simulink model "dynamicsquat_2022a"  (R2022a)
settings: Solver=VariableStepAuto  StartTime=0.0  StopTime=stoptimetotal  RelTol=1e-3
values from neighbouring files (symbols this model uses):
  battery = load('params/battery_Tattu.mat').battery    [runsimulation.m]
  IC = load('params/initialcond/IC_HoverAt30mOcto.mat').IC    [runsimulation.m]
  maxleashvelocity = speed    [runsimulation.m]
  Motor = load('params/KDE4213XF-360_performancedata.mat').Motor    [runsimulation.m]
  motormult = motormults(:)    [runsimulation.m]
  octomodel = load('params/TarotT18.mat').octomodel    [runsimulation.m]
  saturationrpm = saturationrpms(:)    [runsimulation.m]
  scurvetimes = tvec'    [runsimulation.m]
  turbenabled = turb_idx-1    [runsimulation.m]
  velprofileX = qd(1,:)'    [runsimulation.m]
  velprofileY = qd(2,:)'    [runsimulation.m]
  windx = smallestwind + (largestwind-smallestwind)*rand    [runsimulation.m]
  windy = smallestwind + (largestwind-smallestwind)*rand    [runsimulation.m]
  windz = 0    [runsimulation.m]
  xref = xyzref(waypts,1)    [runsimulation.m]
  yref = xyzref(waypts,2)    [runsimulation.m]
undefined symbols (not defined in the file or in its folder): deg, DiscIntNeverNeededParam, F, Light, MIL, rad, s
libraries: aerolibconvert2 x2, shared6dof x1, aerolibwind2 x1
(part 2 of 2)

== system dynamicsquat_2022a/Motors/DC Motor 8/Mechanical part ==
  Static Friction Torque : Inport
  Electrical Torque : Inport  Port=2
  1/J Inertia constant : Gain  Gain=1/Motor.J
  "Df viscous damping coefficient Dynamic Friction coefficient " : Gain  Gain=Motor.Df
  Discrete-Time Integrator : DiscreteIntegrator  gainval=1  InitialCondition=IC.w8  SampleTime=octomodel.sampletime  ICPrevOutput=DiscIntNeverNeededParam  ICPrevScaledInput=DiscIntNeverNeededParam
  Sum1 : Sum  Inputs=--+-
  torque and thrust calculation : Subsystem
  w angular speed : Outport  VectorParamsAs1DForOutWhenUnconnected=off
  Thrust : Outport  Port=2  VectorParamsAs1DForOutWhenUnconnected=off
  Torque : Outport  Port=3  VectorParamsAs1DForOutWhenUnconnected=off
  wires:
  torque and thrust calculation/1(torque) -> Torque/1, Sum1/1
  torque and thrust calculation/2(thrusth) -> Thrust/1
  Electrical Torque/1 -> Sum1/3
  Sum1/1 -> 1/J Inertia constant/1
  Discrete-Time Integrator/1 -> "Df viscous damping coefficient Dynamic Friction coefficient "/1, torque and thrust calculation/1(w angular speed), w angular speed/1  "w angular speed"
  "Df viscous damping coefficient Dynamic Friction coefficient "/1 -> Sum1/4
  Static Friction Torque/1 -> Sum1/2
  1/J Inertia constant/1 -> Discrete-Time Integrator/1

== system dynamicsquat_2022a/Motors/DC Motor 1/Mechanical part/torque and thrust calculation ==
  w angular speed : Inport
  Convert rad/s to rmp : Gain  Gain=60/(2*pi)
  "Propeller model " : MATLAB Function  TreatAsAtomicUnit=on
  torque : Outport  VectorParamsAs1DForOutWhenUnconnected=off
  thrusth : Outport  Port=2  VectorParamsAs1DForOutWhenUnconnected=off
  wires:
  Convert rad/s to rmp/1 -> "Propeller model "/1(rpm)
  w angular speed/1 -> Convert rad/s to rmp/1
  "Propeller model "/2(thrust) -> thrusth/1
  "Propeller model "/1(torque) -> torque/1

== system dynamicsquat_2022a/Motors/DC Motor 2/Mechanical part/torque and thrust calculation ==
  w angular speed : Inport
  Convert rad/s to rmp : Gain  Gain=60/(2*pi)
  "Propeller model " : MATLAB Function  TreatAsAtomicUnit=on
  torque : Outport  VectorParamsAs1DForOutWhenUnconnected=off
  thrusth : Outport  Port=2  VectorParamsAs1DForOutWhenUnconnected=off
  wires:
  "Propeller model "/1(torque) -> torque/1
  "Propeller model "/2(thrust) -> thrusth/1
  w angular speed/1 -> Convert rad/s to rmp/1
  Convert rad/s to rmp/1 -> "Propeller model "/1(rpm)

== system dynamicsquat_2022a/Motors/DC Motor 3/Mechanical part/torque and thrust calculation ==
  w angular speed : Inport
  Convert rad/s to rmp : Gain  Gain=60/(2*pi)
  "Propeller model " : MATLAB Function  TreatAsAtomicUnit=on
  torque : Outport  VectorParamsAs1DForOutWhenUnconnected=off
  thrusth : Outport  Port=2  VectorParamsAs1DForOutWhenUnconnected=off
  wires:
  Convert rad/s to rmp/1 -> "Propeller model "/1(rpm)
  w angular speed/1 -> Convert rad/s to rmp/1
  "Propeller model "/2(thrust) -> thrusth/1
  "Propeller model "/1(torque) -> torque/1

== system dynamicsquat_2022a/Motors/DC Motor 4/Mechanical part/torque and thrust calculation ==
  w angular speed : Inport
  Convert rad/s to rmp : Gain  Gain=60/(2*pi)
  "Propeller model " : MATLAB Function  TreatAsAtomicUnit=on
  torque : Outport  VectorParamsAs1DForOutWhenUnconnected=off
  thrusth : Outport  Port=2  VectorParamsAs1DForOutWhenUnconnected=off
  wires:
  "Propeller model "/1(torque) -> torque/1
  "Propeller model "/2(thrust) -> thrusth/1
  w angular speed/1 -> Convert rad/s to rmp/1
  Convert rad/s to rmp/1 -> "Propeller model "/1(rpm)

== system dynamicsquat_2022a/Motors/DC Motor 5/Mechanical part/torque and thrust calculation ==
  w angular speed : Inport
  Convert rad/s to rmp : Gain  Gain=60/(2*pi)
  "Propeller model " : MATLAB Function  TreatAsAtomicUnit=on
  torque : Outport  VectorParamsAs1DForOutWhenUnconnected=off
  thrusth : Outport  Port=2  VectorParamsAs1DForOutWhenUnconnected=off
  wires:
  Convert rad/s to rmp/1 -> "Propeller model "/1(rpm)
  w angular speed/1 -> Convert rad/s to rmp/1
  "Propeller model "/2(thrust) -> thrusth/1
  "Propeller model "/1(torque) -> torque/1

== system dynamicsquat_2022a/Motors/DC Motor 6/Mechanical part/torque and thrust calculation ==
  w angular speed : Inport
  Convert rad/s to rmp : Gain  Gain=60/(2*pi)
  "Propeller model " : MATLAB Function  TreatAsAtomicUnit=on
  torque : Outport  VectorParamsAs1DForOutWhenUnconnected=off
  thrusth : Outport  Port=2  VectorParamsAs1DForOutWhenUnconnected=off
  wires:
  "Propeller model "/1(torque) -> torque/1
  "Propeller model "/2(thrust) -> thrusth/1
  w angular speed/1 -> Convert rad/s to rmp/1
  Convert rad/s to rmp/1 -> "Propeller model "/1(rpm)

== system dynamicsquat_2022a/Motors/DC Motor 7/Mechanical part/torque and thrust calculation ==
  w angular speed : Inport
  Convert rad/s to rmp : Gain  Gain=60/(2*pi)
  "Propeller model " : MATLAB Function  TreatAsAtomicUnit=on
  torque : Outport  VectorParamsAs1DForOutWhenUnconnected=off
  thrusth : Outport  Port=2  VectorParamsAs1DForOutWhenUnconnected=off
  wires:
  Convert rad/s to rmp/1 -> "Propeller model "/1(rpm)
  w angular speed/1 -> Convert rad/s to rmp/1
  "Propeller model "/2(thrust) -> thrusth/1
  "Propeller model "/1(torque) -> torque/1

== system dynamicsquat_2022a/Motors/DC Motor 8/Mechanical part/torque and thrust calculation ==
  w angular speed : Inport
  Convert rad/s to rmp : Gain  Gain=60/(2*pi)
  "Propeller model " : MATLAB Function  TreatAsAtomicUnit=on
  torque : Outport  VectorParamsAs1DForOutWhenUnconnected=off
  thrusth : Outport  Port=2  VectorParamsAs1DForOutWhenUnconnected=off
  wires:
  "Propeller model "/1(torque) -> torque/1
  "Propeller model "/2(thrust) -> thrusth/1
  w angular speed/1 -> Convert rad/s to rmp/1
  Convert rad/s to rmp/1 -> "Propeller model "/1(rpm)

== matlab function dynamicsquat_2022a/Motors/DC Motor 8/Mechanical part/torque and thrust calculation/Propeller model  ==
  data: torque output; rpm input; thrust output
function [torque,thrust] = fcn(rpm)
%% Tarot model data

%coefficient of thrust, empirically derived
coef_t = 0.065;
%thrust = coef_t * density of air * velocity^2 * propeller diameter (m) ^4
%velocity in rev/sec, where  1 rev/sec = 1 rpm/60
thrust = coef_t*1.225*(rpm/60)^2*.47^4; % 18.5 inches ~ 0.47 m
% empirically derived
torque = (2.138e-08)*rpm^2 + (-1.279e-05)*rpm ;% (0.0216);

end

== matlab function dynamicsquat_2022a/arrival condition ==
  data: currentpos input; arrived output; dest input
function arrived = fcn(currentpos,dest)
result=norm(currentpos-dest);
if result<2 % less than one meter from the goal
    arrived=1;
else
    arrived=0;
end

== matlab function dynamicsquat_2022a/Power Consumption Calculation ==
  data: DC input; tot_mot_i output; Imot input
function tot_mot_i  = fcn(DC,Imot)
imot=zeros(8,1);
for i=1:length(DC)
    imot(i)=DC(i)*Imot(i);
end
tot_mot_i=sum(imot);
tot_mot_i=sum(Imot);
end

== matlab function dynamicsquat_2022a/Drag Force and Moment Calculation ==
  data: Vw_nom input; Fdrag output; Vw_turb input; Vb input; wb input; Mdrag output; Eul input; windspecs parameter
function [Fdrag,Mdrag]  = fcn(Vw_nom,Vw_turb,Vb,wb,Eul, windspecs)
%% Parameters 
% windspecs - airframe wind-related specs
% Vw_nom - nominal wind velocity in m/s in inertial frame
% Vw_turb - turbulence wind velocity in m/s in inertial frame
% Vb - linear velocity body frame
% wb - angular velocity body frame
% Eul - Euler angles inertial frame
model = windspecs;

% Z-Y-X rotation convention 
Phi = Eul(1);
The = Eul(2);
Psi = Eul(3);
R_b_e = [cos(Psi)*cos(The) cos(Psi)*sin(The)*sin(Phi)-sin(Psi)*cos(Phi) cos(Psi)*sin(The)*cos(Phi)+sin(Psi)*sin(Phi);
       sin(Psi)*cos(The) sin(Psi)*sin(The)*sin(Phi)+cos(Psi)*cos(Phi) sin(Psi)*sin(The)*cos(Phi)-cos(Psi)*sin(Phi);
       -sin(The)         cos(The)*sin(Phi)                            cos(The)*cos(Phi)]; % Rib
R_e_b = R_b_e'; % Rbi  

% 3-torque created by drag
p = wb(1);
q = wb(2);
r = wb(3);
Mdrag=(((-1/2)*model.rho*model.cd)*[model.Axy*p*abs(p)*model.lx model.Axy*q*abs(q)*model.ly 8*model.Ayz*r*abs(r)*model.lz])';

% Wind in the inertial frame

v_we=Vw_nom+Vw_turb; % wind velocity in m/s in inertial frame
v_wb=R_e_b*v_we; % wind velocity in m/s in body frame
v_a=v_wb+Vb; % apparent velocity resulting from wind and body

% 3-Drag force
Fdrag=(((-1/2)*model.rho*model.cd)*[model.Ayz*v_a(1)*abs(v_a(1)) model.Axz*v_a(2)*abs(v_a(2)) model.Axy*v_a(3)*abs(v_a(3))])';


end

== matlab function dynamicsquat_2022a/Adding position//velocity noise ==
  data: u input; y output
function y = fcn(u)

y = zeros(6,1);
posnoisestd=0.75; % gives maximum and minimum of +-3 meters
velnoisestd=0.025;
noisepos=posnoisestd.*randn(3,1);
noisevel=velnoisestd.*randn(3,1);
noise=[noisepos ;noisevel];
y = y + u + noise;

== matlab function dynamicsquat_2022a/Position//Velocity controllers/Ref Velocity Calculation ==
  data: reference input; ref_velx output double size=1; measurement input; yaw input; ref_vely output double size=1; errprev input size=[2 1]; errprev output; maxspeed input; scurvevelX input; scurvevelY input; scurvetimes input; time input; Xdot input; Ydot input
function [ref_velx,ref_vely,errprev] = fcn(reference,measurement,yaw,errprev,maxspeed,scurvevelX,scurvevelY,scurvetimes,time,Xdot,Ydot)
%% parameters
k_p=0.5;
k_d=0.05;%ki=;
dt=0.01; %controller frequency
max_velocity=maxspeed;% m/s
if scurvevelX(1)>0
    see=1;
end

%% output calculation

err = reference - measurement;
err_len = norm(err);

% calculate desired velocity for each axis

err_p = k_p * err;
% err_i = self.k_i * np.clip(
%     self.err_i + trapezoid((self.err, err), dx=self.dt, axis=0),
%     a_min=-self.max_err_i, a_max=self.max_err_i
% )
err_d = k_d * (err - errprev) / dt;
%direct velocity usage
velerr=[Xdot,Ydot]';
err_d2 = k_d * velerr;
velocity = err_p ;%+ err_d2;%+ self.err_i ;


% if self.leashing:
%     err_unit = err / (err_len + 1e-6)
%     err_len = min(err_len, self.leash)
%     err = err_unit * err_len
%     self.err = err
%     velocity = self.err_p = self.k_p * err
% if err_len > 0. and self.square_root_scaling:
%     velocity = np.zeros_like(self.k_p)
%     velocity[0] = sqrt_control(err[0], self.k_p[0], self.max_acceleration, self.dt)
%     velocity[1] = sqrt_control(err[1], self.k_p[1], self.max_acceleration, self.dt)
%     # scale velocity correction by error size
%     # velocity = (np.abs(err) / err_len) * velocity
%     self.err = err
%     self.err_p = velocity
% else:
%    velocity = super().step(reference, measurement)


% convert to body-frame velocity
%yaw=0;
rot = [cos(yaw)   sin(yaw); ...
    -sin(yaw) cos(yaw)];
ref_velocity = rot * velocity; % velocity is a row vector [vx, vy]

%compute abs max velocity allowed based on max_velocity - Ibrahim's
%implementation
%abs_max_vel = abs((ref_velocity/(norm(ref_velocity)+ 1e-6))* max_velocity);
%clip velocity values according to max allowed
% if (ref_velocity>abs_max_vel)
%     ref_velocity(ref_velocity>abs_max_vel)=abs_max_vel(ref_velocity>abs_max_vel);%ref_velocity = abs_max_vel;
% elseif(ref_velocity<-abs_max_vel)
%     ref_velocity(ref_velocity<-abs_max_vel)=abs_max_vel(ref_velocity<-abs_max_vel);%ref_velocity = -abs_max_vel;
% end

% constraint max velocity v1
if abs(norm(ref_velocity)+ 1e-6)>max_velocity
    % preserve direction but constraint total velocity to max
    ref_velocity=(ref_velocity/norm(ref_velocity)+ 1e-6)* max_velocity;
end


%weigthed average of position controller velocity and s-curve based
%velocity
wpos=[0.5 0.5];%wpos=[0.8 0.8];
wscurve=[0.5 0.5];%wscurve=[0.2 0.2];
%[index, ~]=find(scurvetimes==interp1(scurvetimes,scurvetimes,time,'nearest'),1,'first');
index=scurvetimes==interp1(scurvetimes,scurvetimes,time,'nearest');

value=time;
array=scurvetimes;
cur = abs(array-value);
% df is the minimum distance, ind is the index of the minimum distance
[df,ind] = min(cur);  


scurvepartX = zeros(1,1);scurvepartX = scurvevelX(ind);
scurvepartY=zeros(1,1);scurvepartY=scurvevelY(ind);
% dummyx=zeros(1,1);dummyy=zeros(1,1);
% dummyx=wpos(1)*ref_velocity(1)+wscurve(1)*scurvepartX;
% dummyy=wpos(2)*ref_velocity(2)+wscurve(2)*scurvepartY; 
% ref_velx=zeros(1,1);ref_vely=zeros(1,1);

if scurvevelX(ind)>2
    see=1;
end
 ref_velx=wpos(1)*ref_velocity(1)+wscurve(1)*scurvepartX;
 ref_vely=wpos(2)*ref_velocity(2)+wscurve(2)*scurvepartY;   
%   ref_velx=scurvepartX;
%   ref_vely=scurvepartY;  
%  ref_velx=ref_velocity(1);
%  ref_vely=ref_velocity(2);  

errprev=err;

== matlab function dynamicsquat_2022a/Motors/DC Motor 1/Mechanical part/torque and thrust calculation/Propeller model  ==
  data: torque output; rpm input; thrust output
function [torque,thrust] = fcn(rpm)
%% Tarot model data

%coefficient of thrust, empirically derived
coef_t = 0.065;
%thrust = coef_t * density of air * velocity^2 * propeller diameter (m) ^4
%velocity in rev/sec, where  1 rev/sec = 1 rpm/60
thrust = coef_t*1.225*(rpm/60)^2*.47^4; % 18.5 inches ~ 0.47 m
% empirically derived
torque = (2.138e-08)*rpm^2 + (-1.279e-05)*rpm ;% (0.0216);

end

== matlab function dynamicsquat_2022a/Forces and Moments Calculation ==
  data: w1 input; Fx output; w2 input; w3 input; w4 input; w5 input; w6 input; Fy output; Fz output; Mx output; My output; Mz output; w7 input; w8 input; Phi input; The input; Psi input
function [Fx,Fy,Fz,Mx,My,Mz] = fcn(w1,w2,w3,w4,w5,w6,w7,w8,Phi,The,Psi)
octomodel.g=9.80;
octomodel.m_t=10.66;
octomodel.l=0.635;
% Phi,The,Psi, in rad
w  = [w1; w2; w3; w4;w5; w6; w7; w8];

%% not used
%to fix numerical issues
%w=round(w,2);
% transform rpm to rad/s
%w=w./(60/(2*pi));

%% thrust generated by rotors

% Approach 1
% coef_t = 0.065;
%thrust = coef_t * density of air * velocity^2 * propeller diameter (m) ^4
%velocity in rev/sec, where  1 rev/sec = 1 rpm/60
%T = coef_t*1.225*((w./60).^2)*.47^4; % 18.5 inches ~ 0.47 m

% Approach 2
% thrust motor constant [Ns^2/rad^2]
b=9.8419e-05; % 
T = b.*((2*pi).*w./60).^2;

% total thrust generated by rotors
T_total=sum(T);
T_total=round(T_total*100)/100;

%% Forces in the local frame 
R_b_e = [cos(Psi)*cos(The) cos(Psi)*sin(The)*sin(Phi)-sin(Psi)*cos(Phi) cos(Psi)*sin(The)*cos(Phi)+sin(Psi)*sin(Phi);
       sin(Psi)*cos(The) sin(Psi)*sin(The)*sin(Phi)+cos(Psi)*cos(Phi) sin(Psi)*sin(The)*cos(Phi)-cos(Psi)*sin(Phi);
       -sin(The)         cos(The)*sin(Phi)                            cos(The)*cos(Phi)]; % Rib

Ftot_b=R_b_e'*[0 ;0; -octomodel.m_t*octomodel.g]+[0; 0; T_total]; 
Fx=Ftot_b(1);Fy=Ftot_b(2);Fz=Ftot_b(3);

%% Moments in the local frame 
% moment of each rotor
% Approach 1
%M = (2.138e-08)*w.^2 + (-1.279e-05)*w ;

% Approach 2
% rotor drag constant [Nms^2/rad^2]
d=1.8503e-06; % 
M = d.*((2*pi).*w./60).^2;


% torque generated by rotors
%motor angles
angsm=cos(pi/8); % 22.5 
anglg=cos(3*pi/8); % 67.5

Mx=octomodel.l*(T(1)*anglg +T(2)*angsm -T(3)*angsm -T(4)*anglg -T(5)*anglg ...
    -T(6)*angsm +T(7)*angsm +T(8)*anglg);%Tau_roll

My=octomodel.l*(-T(1)*angsm -T(2)*anglg -T(3)*anglg -T(4)*angsm +T(5)*angsm ...
    +T(6)*anglg +T(7)*anglg +T(8)*angsm);%Tau_theta

Mz= M(1) -M(2) +M(3) -M(4) +M(5) -M(6) +M(7) -M(8);%%Tau_yaw
end

== matlab function dynamicsquat_2022a/Motors/DC Motor 2/Mechanical part/torque and thrust calculation/Propeller model  ==
  data: torque output; rpm input; thrust output
function [torque,thrust] = fcn(rpm)
%% Tarot model data

%coefficient of thrust, empirically derived
coef_t = 0.065;
%thrust = coef_t * density of air * velocity^2 * propeller diameter (m) ^4
%velocity in rev/sec, where  1 rev/sec = 1 rpm/60
thrust = coef_t*1.225*(rpm/60)^2*.47^4; % 18.5 inches ~ 0.47 m
% empirically derived
torque = (2.138e-08)*rpm^2 + (-1.279e-05)*rpm ;% (0.0216);

end

== matlab function dynamicsquat_2022a/Motors/DC Motor 3/Mechanical part/torque and thrust calculation/Propeller model  ==
  data: torque output; rpm input; thrust output
function [torque,thrust] = fcn(rpm)
%% Tarot model data

%coefficient of thrust, empirically derived
coef_t = 0.065;
%thrust = coef_t * density of air * velocity^2 * propeller diameter (m) ^4
%velocity in rev/sec, where  1 rev/sec = 1 rpm/60
thrust = coef_t*1.225*(rpm/60)^2*.47^4; % 18.5 inches ~ 0.47 m
% empirically derived
torque = (2.138e-08)*rpm^2 + (-1.279e-05)*rpm ;% (0.0216);

end

== matlab function dynamicsquat_2022a/Motors/DC Motor 4/Mechanical part/torque and thrust calculation/Propeller model  ==
  data: torque output; rpm input; thrust output
function [torque,thrust] = fcn(rpm)
%% Tarot model data

%coefficient of thrust, empirically derived
coef_t = 0.065;
%thrust = coef_t * density of air * velocity^2 * propeller diameter (m) ^4
%velocity in rev/sec, where  1 rev/sec = 1 rpm/60
thrust = coef_t*1.225*(rpm/60)^2*.47^4; % 18.5 inches ~ 0.47 m
% empirically derived
torque = (2.138e-08)*rpm^2 + (-1.279e-05)*rpm ;% (0.0216);

end

== matlab function dynamicsquat_2022a/Motors/DC Motor 5/Mechanical part/torque and thrust calculation/Propeller model  ==
  data: torque output; rpm input; thrust output
function [torque,thrust] = fcn(rpm)
%% Tarot model data

%coefficient of thrust, empirically derived
coef_t = 0.065;
%thrust = coef_t * density of air * velocity^2 * propeller diameter (m) ^4
%velocity in rev/sec, where  1 rev/sec = 1 rpm/60
thrust = coef_t*1.225*(rpm/60)^2*.47^4; % 18.5 inches ~ 0.47 m
% empirically derived
torque = (2.138e-08)*rpm^2 + (-1.279e-05)*rpm ;% (0.0216);

end

== matlab function dynamicsquat_2022a/Motors/DC Motor 6/Mechanical part/torque and thrust calculation/Propeller model  ==
  data: torque output; rpm input; thrust output
function [torque,thrust] = fcn(rpm)
%% Tarot model data

%coefficient of thrust, empirically derived
coef_t = 0.065;
%thrust = coef_t * density of air * velocity^2 * propeller diameter (m) ^4
%velocity in rev/sec, where  1 rev/sec = 1 rpm/60
thrust = coef_t*1.225*(rpm/60)^2*.47^4; % 18.5 inches ~ 0.47 m
% empirically derived
torque = (2.138e-08)*rpm^2 + (-1.279e-05)*rpm ;% (0.0216);

end

== matlab function dynamicsquat_2022a/Motors/DC Motor 7/Mechanical part/torque and thrust calculation/Propeller model  ==
  data: torque output; rpm input; thrust output
function [torque,thrust] = fcn(rpm)
%% Tarot model data

%coefficient of thrust, empirically derived
coef_t = 0.065;
%thrust = coef_t * density of air * velocity^2 * propeller diameter (m) ^4
%velocity in rev/sec, where  1 rev/sec = 1 rpm/60
thrust = coef_t*1.225*(rpm/60)^2*.47^4; % 18.5 inches ~ 0.47 m
% empirically derived
torque = (2.138e-08)*rpm^2 + (-1.279e-05)*rpm ;% (0.0216);

end

== matlab function dynamicsquat_2022a/Control allocation ==
  data: Fx input; wref1 output; Fy input; Fz input; Troll input; Tpitch input; Tyaw input; wref2 output; wref3 output; wref4 output; wref5 output; wref6 output; wref7 output; wref8 output; Vbat input; DC output
function [wref1,wref2,wref3,wref4,wref5,wref6,wref7,wref8,DC] = fcn(Fx,Fy,Fz,Troll,Tpitch,Tyaw,Vbat)
%% parameters 
%Maximum speed that the motors can reach in rad/s
Max_speed=670; %668.11
%Max total Thrust all motors can generate in N
Max_thrust=352; %351.451
%Max torque in each individual axis



% arm length - distances from the octorotor center of mass ...
%        to the center of mass of all its rotors are equal and denoted by l.
l=0.635;
% thrust motor constant [Ns^2/rad^2]
b=9.8419e-05; % 
% rotor drag constant [Nms^2/rad^2]
d=1.8503e-06; % 

%angles
angsm=cos(pi/8); % 22.5 
anglg=cos(3*pi/8); % 67.5

% control allocation matrix
A_f=[b b b b b b b b; ...
    b*l*anglg b*l*angsm -b*l*angsm -b*l*anglg -b*l*anglg -b*l*angsm b*l*angsm b*l*anglg; ...
    -b*l*angsm -b*l*anglg -b*l*anglg -b*l*angsm b*l*angsm b*l*anglg b*l*anglg b*l*angsm; ...
    d -d d -d d -d d -d];

% duty cycle initialization
DC=zeros(8,1);

%desired input
u_des=[Fz;Troll;Tpitch;Tyaw];

%control allocation
Omega_s=pinv(A_f)*u_des; %inverse of A_f is A_f\

% velocity checking
wref=zeros(8,1);
for i=1:length(Omega_s)
    if Omega_s(i)<0
        wref(i)=0;
    elseif Omega_s(i)>Max_speed^2
        wref(i)=Max_speed;
    else
        wref(i)=sqrt(Omega_s(i));
    end
end

%velocity assignment in V
DCfactor=0.001355; %original direct conversion multiply=0.0325; wref(i)=wref(i)*multiply;
Voltconversion=0.0325;

% "virtual" ESC 
for i=1:length(wref)
    % voltage saturation check
    if(wref(i)*DCfactor*Vbat > Vbat)
        wref(i)=Vbat;
        DC(i)=1;
    elseif(wref(i)*DCfactor*Vbat <=0)
        wref(i)=0.065;
        DC(i)=0.01;
    else
        DC(i)=wref(i)*DCfactor;
        %wref(i)=Vbat*DC(i); 
        wref(i)=wref(i)*Voltconversion;
    end
end

wref1=wref(1);
wref2=wref(2);
wref3=wref(3);
wref4=wref(4);
wref5=wref(5);
wref6=wref(6);
wref7=wref(7);
wref8=wref(8);


end
